simulink model "sfcndemo_vsfunc"  (Simulink 6.0)
settings: Solver=ode45  StartTime=0.0  StopTime=50  RelTol=1e-3
settings Model: Creator=The MathWorks Inc.  LastModifiedBy=batserve  ExtModeTrigMode=oneshot  ExtModeArmWhenConnect=off  ExtModeAutoUpdateStatusClock=off
settings DataIOCC: LimitDataPoints=off  SaveFormat=StructureWithTime  SaveState=on  OutputSaveName=yout1
settings OptimizationCC: BlockReduction=off  BooleanDataType=off
settings DebuggingCC: CheckExecutionContextPreStartOutputMsg=on  CheckExecutionContextRuntimeOutputMsg=on  SolverPrmCheckMsg=none
settings HardwareCC: TargetUnknown=on

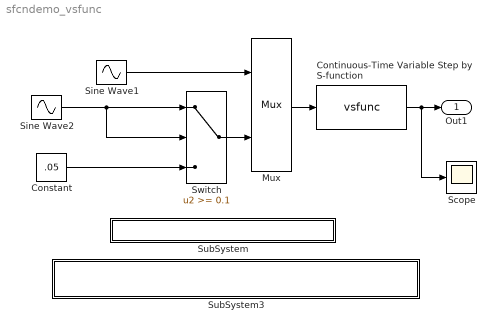
== system sfcndemo_vsfunc ==
  Constant : Constant  Value=.05
  Continuous-Time Variable Step by S-function : S-Function  FunctionName=vsfunc
      mask Display: disp('dt           = u(2)\ny(t + dt) = u(t)')
  Mux : Mux  Inputs=2
  Scope : Scope
      settings: TimeRange=10  YMin=-1.6e-15  YMax=0  SaveName=scopeout1
  Sine Wave1 : Sin  Frequency=2*pi  SampleTime=0
  Sine Wave2 : Sin  Amplitude=2  Frequency=2*pi  SampleTime=0
  SubSystem : Subsystem  PropExecContextAcrossSSBoundary=on
      settings: OpenFcn=edit(fullfile(matlabroot,'simulink','src','vsfunc.c'))
      mask Display: disp('matlabroot\simulink\src\vsfunc.c');
  SubSystem3 : Subsystem  PropExecContextAcrossSSBoundary=on
      settings: OpenFcn=edit(fullfile(matlabroot,'toolbox','simulink','blocks','vsfunc.m'))
      mask Display: disp('M-file: matlabroot\toolbox\simulink\blocks\vsfunc.m\nNote:to run the m-file, please disable the executable mex file in your path.');
  Switch : Switch  Threshold=0.1  SaturateOnIntegerOverflow=on  InputSameDT=on
  Out1 : Outport  InitialOutput=0
  wires:
  Constant/1 -> Switch/3
  Mux/1 -> Continuous-Time Variable Step by S-function/1
  Sine Wave2/1 -> Switch/1, Switch/2
  Continuous-Time Variable Step by S-function/1 -> Out1/1, Scope/1
  Sine Wave1/1 -> Mux/1
  Switch/1 -> Mux/2

== system sfcndemo_vsfunc/SubSystem ==

== system sfcndemo_vsfunc/SubSystem3 ==
